simulink model "PIDPitch"  (R2012b)
settings: Solver=ode45  StartTime=0.0  StopTime=40.0  RelTol=1e-3
undefined symbols (not defined in the file): DiscIntNeverNeededParam, Ts
libraries: simulink x1, slident x1
settings Model: Creator=TOSHIBA  LastModifiedBy=Carlos

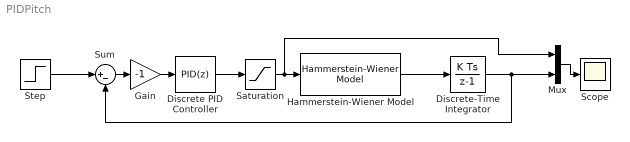
== system PIDPitch ==
  Discrete PID Controller : simulink/Continuous/PID Controller  Controller=PID  TimeDomain=Discrete-time  SampleTime=Ts  IntegratorMethod=Forward Euler  FilterMethod=Forward Euler  Form=Parallel  P=0.7  I=0  D=0.5  N=15  InitialConditionSource=internal  InitialConditionForIntegrator=0  InitialConditionForFilter=0  ExternalReset=none  LimitOutput=off  UpperSaturationLimit=inf  LowerSaturationLimit=-inf  LinearizeAsGain=off  AntiWindupMode=none  Kb=1  TrackingMode=off  Kt=1  PParamMin=[]  PParamMax=[]  IParamMin=[]  IParamMax=[]  DParamMin=[]  DParamMax=[]  NParamMin=[]  NParamMax=[]  KbParamMin=[]  KbParamMax=[]  KtParamMin=[]  KtParamMax=[]  POutMin=[]  POutMax=[]  IOutMin=[]  IOutMax=[]  DOutMin=[]  DOutMax=[]  NOutMin=[]  NOutMax=[]  KbOutMin=[]  KbOutMax=[]  KtOutMin=[]  KtOutMax=[]  IntegratorOutMin=[]  IntegratorOutMax=[]  FilterOutMin=[]  FilterOutMax=[]  SumOutMin=[]  SumOutMax=[]  SumI1OutMin=[]  SumI1OutMax=[]  SumI2OutMin=[]  SumI2OutMax=[]  SumI3OutMin=[]  SumI3OutMax=[]  SumDOutMin=[]  SumDOutMax=[]  SaturationOutMin=[]  SaturationOutMax=[]  IntegratorContinuousStateAttributes=''  IntegratorStateMustResolveToSignalObject=off  IntegratorRTWStateStorageClass=Auto  FilterContinuousStateAttributes=''  FilterStateMustResolveToSignalObject=off  FilterRTWStateStorageClass=Auto
  Discrete-Time Integrator : DiscreteIntegrator  SampleTime=Ts  ICPrevOutput=DiscIntNeverNeededParam  ICPrevScaledInput=DiscIntNeverNeededParam
  Gain : Gain  Gain=-1  SampleTime=Ts
  Hammerstein-Wiener Model : slident/Hammerstein-Wiener Model  sys=vx123_nlhw113_pic2  IC=Zero  X0i=0
  Mux : Mux  Inputs=2
  Saturation : Saturate  SampleTime=Ts
  Scope : Scope
  Step : Step  After=1.2  SampleTime=0
  Sum : Sum  Inputs=|+-
  wires:
  Hammerstein-Wiener Model/1 -> Discrete-Time Integrator/1
  Step/1 -> Sum/1
  Discrete-Time Integrator/1 -> Sum/2, Mux/2
  Sum/1 -> Gain/1
  Gain/1 -> Discrete PID Controller/1
  Saturation/1 -> Mux/1, Hammerstein-Wiener Model/1
  Mux/1 -> Scope/1
  Discrete PID Controller/1 -> Saturation/1
